simulink model "AERO421_FP4"  (R2024b)
settings: Solver=ode45  StartTime=0.0  StopTime=tspan  RelTol=1e-8  AbsTol=1e-8
model workspace (MATLAB code in the model file):
  | mu = 398601; % km
  | Re = 6378.137; %km
values from neighbouring files (symbols this model uses):
  E_b_ECI_0 = C2EulerAngles(C_b_ECI_0)    [AERO421_FP4_RJF_SR.m]
  E_b_LVLH_0 = [phi_0; theta_0; psi_0]    [AERO421_FP4_RJF_SR.m]
  q_b_ECI_0 = rotm2quat(C_b_ECI_0)    [AERO421_FP4_RJF_SR.m]
  q_b_LVLH_0 = [0; 0; 0; 1]    [AERO421_FP4_RJF_SR.m]
  T_c = [0; 0; 0]    [AERO421_FP4_RJF_SR.m]
  w_b_ECI_0 = [0.001; -0.001; 0.002]    [AERO421_FP4_RJF_SR.m]
undefined symbols (not defined in the file or in its folder): J, r_ECI_0, v_ECI_0
settings Model: Creator=emehiel  LastModifiedBy=rosha
settings SolverCC: AlgebraicLoopSolver=TrustRegion
settings DebuggingCC: UnconnectedInputMsg=warning  UnconnectedOutputMsg=warning  UnconnectedLineMsg=warning
settings ModelReferenceCC: EnableRefExpFcnMdlSchedulingChecks=on
settings RTWCC: GPUComputeCapability=3.5

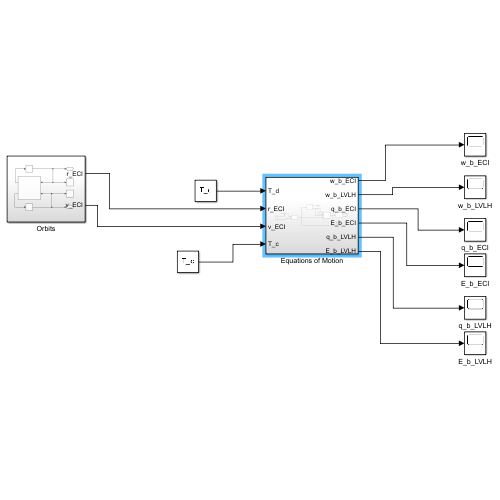
[thumbnail: Simulink's stored preview of the top-level diagram]
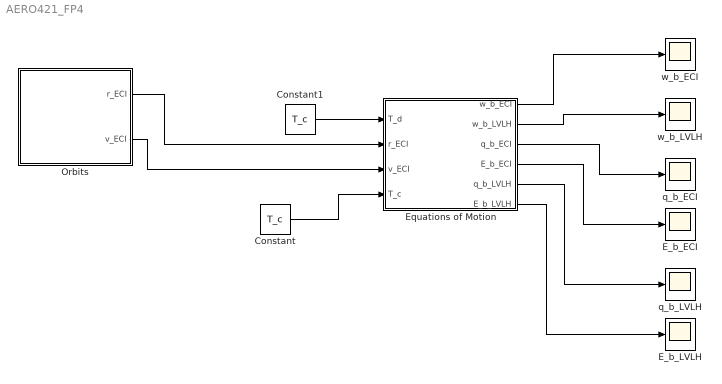
== system AERO421_FP4 ==
  Constant : Constant  Value=T_c
  Constant1 : Constant  Value=T_c
  E_b_ECI : Scope
  E_b_LVLH : Scope
  Equations of Motion : Subsystem
  Orbits : Subsystem
  q_b_ECI : Scope
  q_b_LVLH : Scope
  w_b_ECI : Scope
  w_b_LVLH : Scope
  wires:
  Orbits/1(r_ECI) -> Equations of Motion/2(r_ECI)
  Equations of Motion/3(q_b_ECI) -> q_b_ECI/1
  Equations of Motion/1(w_b_ECI) -> w_b_ECI/1
  Equations of Motion/4(E_b_ECI) -> E_b_ECI/1
  Equations of Motion/2(w_b_LVLH) -> w_b_LVLH/1
  Equations of Motion/5(q_b_LVLH) -> q_b_LVLH/1
  Equations of Motion/6(E_b_LVLH) -> E_b_LVLH/1
  Orbits/2(v_ECI) -> Equations of Motion/3(v_ECI)
  Constant/1 -> Equations of Motion/4(T_c)
  Constant1/1 -> Equations of Motion/1(T_d)

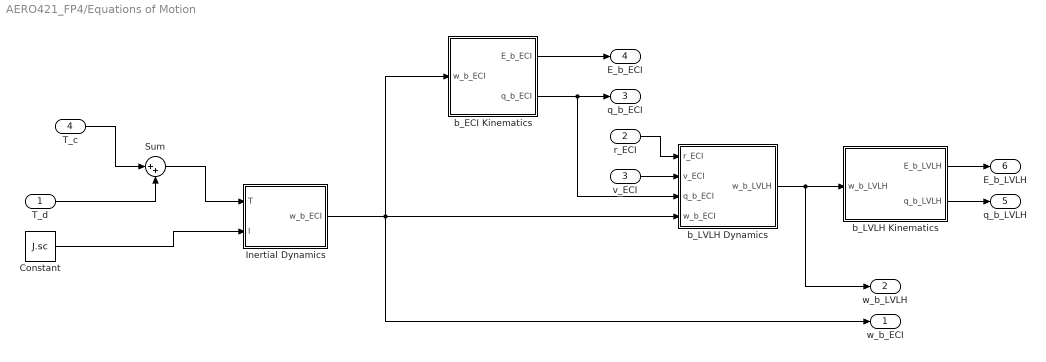
== system AERO421_FP4/Equations of Motion ==
  T_d : Inport
  r_ECI : Inport  Port=2
  v_ECI : Inport  Port=3
  T_c : Inport  Port=4
  Constant : Constant  Value=J.sc
  Inertial Dynamics : Subsystem
  Sum : Sum  Inputs=|++
  b_ECI Kinematics : Subsystem
  b_LVLH Dynamics : Subsystem
  b_LVLH Kinematics : Subsystem
  w_b_ECI : Outport  VectorParamsAs1DForOutWhenUnconnected=off
  w_b_LVLH : Outport  Port=2  PortDimensions=[3 1]  VectorParamsAs1DForOutWhenUnconnected=off
  q_b_ECI : Outport  Port=3  PortDimensions=[4 1]  VectorParamsAs1DForOutWhenUnconnected=off
  E_b_ECI : Outport  Port=4  PortDimensions=[3 1]  VectorParamsAs1DForOutWhenUnconnected=off
  q_b_LVLH : Outport  Port=5  PortDimensions=[4 1]  VectorParamsAs1DForOutWhenUnconnected=off
  E_b_LVLH : Outport  Port=6  PortDimensions=[3 1]  VectorParamsAs1DForOutWhenUnconnected=off
  wires:
  b_ECI Kinematics/1(E_b_ECI) -> E_b_ECI/1
  Constant/1 -> Inertial Dynamics/2(I)
  b_LVLH Kinematics/1(E_b_LVLH) -> E_b_LVLH/1
  Inertial Dynamics/1(w_b_ECI) -> w_b_ECI/1, b_ECI Kinematics/1(w_b_ECI), b_LVLH Dynamics/4(w_b_ECI)
  b_ECI Kinematics/2(q_b_ECI) -> b_LVLH Dynamics/3(q_b_ECI), q_b_ECI/1
  b_LVLH Kinematics/2(q_b_LVLH) -> q_b_LVLH/1
  r_ECI/1 -> b_LVLH Dynamics/1("r_ECI ")
  v_ECI/1 -> b_LVLH Dynamics/2(v_ECI)
  b_LVLH Dynamics/1(w_b_LVLH) -> w_b_LVLH/1, b_LVLH Kinematics/1(w_b_LVLH)
  T_d/1 -> Sum/2
  T_c/1 -> Sum/1
  Sum/1 -> Inertial Dynamics/1(T)

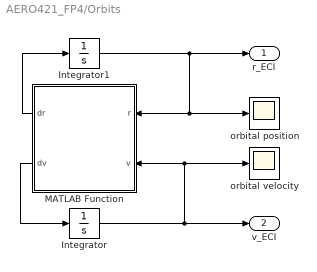
== system AERO421_FP4/Orbits ==
  Integrator : Integrator  InitialCondition=v_ECI_0
  Integrator1 : Integrator  InitialCondition=r_ECI_0
  MATLAB Function : MATLAB Function  TreatAsAtomicUnit=on
  orbital position : Scope
  orbital velocity : Scope
  r_ECI : Outport  VectorParamsAs1DForOutWhenUnconnected=off
  v_ECI : Outport  Port=2  VectorParamsAs1DForOutWhenUnconnected=off
  wires:
  Integrator/1 -> orbital velocity/1, MATLAB Function/2(v), v_ECI/1
  Integrator1/1 -> orbital position/1, MATLAB Function/1(r), r_ECI/1
  MATLAB Function/1(dr) -> Integrator1/1
  MATLAB Function/2(dv) -> Integrator/1

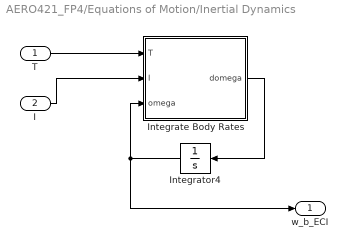
== system AERO421_FP4/Equations of Motion/Inertial Dynamics ==
  T : Inport
  I : Inport  Port=2
  Integrate Body Rates : MATLAB Function  TreatAsAtomicUnit=on
  Integrator4 : Integrator  InitialCondition=w_b_ECI_0
  w_b_ECI : Outport  VectorParamsAs1DForOutWhenUnconnected=off
  wires:
  Integrate Body Rates/1(domega) -> Integrator4/1
  I/1 -> Integrate Body Rates/2(I)
  T/1 -> Integrate Body Rates/1(T)
  Integrator4/1 -> w_b_ECI/1, Integrate Body Rates/3(omega)

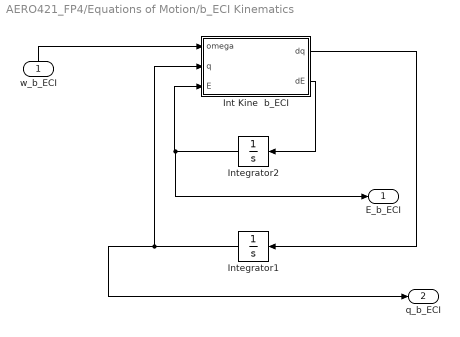
== system AERO421_FP4/Equations of Motion/b_ECI Kinematics ==
  w_b_ECI : Inport
  Int Kine  b_ECI : MATLAB Function  TreatAsAtomicUnit=on
  Integrator1 : Integrator  InitialCondition=q_b_ECI_0
  Integrator2 : Integrator  InitialCondition=E_b_ECI_0
  E_b_ECI : Outport  PortDimensions=[3 1]  VectorParamsAs1DForOutWhenUnconnected=off
  q_b_ECI : Outport  Port=2  PortDimensions=[4 1]  VectorParamsAs1DForOutWhenUnconnected=off
  wires:
  w_b_ECI/1 -> Int Kine  b_ECI/1(omega)
  Int Kine  b_ECI/1(dq) -> Integrator1/1
  Int Kine  b_ECI/2(dE) -> Integrator2/1
  Integrator1/1 -> q_b_ECI/1, Int Kine  b_ECI/2(q)
  Integrator2/1 -> E_b_ECI/1, Int Kine  b_ECI/3(E)

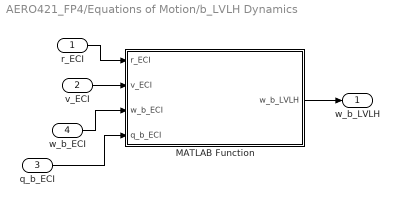
== system AERO421_FP4/Equations of Motion/b_LVLH Dynamics ==
  "r_ECI " : Inport
  v_ECI : Inport  Port=2
  q_b_ECI : Inport  Port=3
  w_b_ECI : Inport  Port=4
  MATLAB Function : MATLAB Function  TreatAsAtomicUnit=on
  w_b_LVLH : Outport  VectorParamsAs1DForOutWhenUnconnected=off
  wires:
  MATLAB Function/1(w_b_LVLH) -> w_b_LVLH/1
  "r_ECI "/1 -> MATLAB Function/1(r_ECI)
  v_ECI/1 -> MATLAB Function/2(v_ECI)
  q_b_ECI/1 -> MATLAB Function/4(q_b_ECI)
  w_b_ECI/1 -> MATLAB Function/3(w_b_ECI)

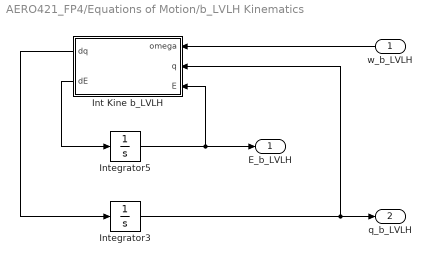
== system AERO421_FP4/Equations of Motion/b_LVLH Kinematics ==
  w_b_LVLH : Inport
  Int Kine b_LVLH : MATLAB Function  TreatAsAtomicUnit=on
  Integrator3 : Integrator  InitialCondition=q_b_LVLH_0
  Integrator5 : Integrator  InitialCondition=E_b_LVLH_0
  E_b_LVLH : Outport  PortDimensions=[3 1]  VectorParamsAs1DForOutWhenUnconnected=off
  q_b_LVLH : Outport  Port=2  VectorParamsAs1DForOutWhenUnconnected=off
  wires:
  Int Kine b_LVLH/1(dq) -> Integrator3/1
  Integrator3/1 -> Int Kine b_LVLH/2(q), q_b_LVLH/1
  Int Kine b_LVLH/2(dE) -> Integrator5/1
  Integrator5/1 -> E_b_LVLH/1, Int Kine b_LVLH/3(E)
  w_b_LVLH/1 -> Int Kine b_LVLH/1(omega)

== matlab function AERO421_FP4/Equations of Motion/Inertial Dynamics/Integrate Body Rates ==
  data: T input; I input; omega input; domega output
function domega = dynamics(T, I, omega)
%#codegen

domega = I\(T - cross(omega, I*omega));

== matlab function AERO421_FP4/Equations of Motion/b_ECI Kinematics/Int Kine  b_ECI ==
  data: omega input; q input; dq output; E input; dE output
function [dq,dE] = kinematics(omega, q, E)
%#codegen

% unpack quaternion

epsilon = q(1:3,1);
eta = q(4,1);

depsilon = 1/2*(eta*eye(3) + vcross(epsilon))*omega;
deta = -1/2*epsilon'*omega;

dq = [depsilon; deta];

LBI = 1/cos(E(2))*[cos(E(2)) sin(E(1))*sin(E(2))  cos(E(1))*sin(E(2));
                   0         cos(E(1))*cos(E(2)) -sin(E(1))*cos(E(2));
                   0         sin(E(1))            cos(E(1))];

dE = LBI*omega;

== matlab function AERO421_FP4/Orbits/MATLAB Function ==
  data: r input; dr output; v input; dv output
function [dr,dv] = orbitalDynamics(r, v)
%#codegen

mu = 398601; % km^3/s^2

dr = v;
dv = -mu*r/norm(r)^3;

== matlab function AERO421_FP4/Equations of Motion/b_LVLH Dynamics/MATLAB Function ==
  data: r_ECI input; v_ECI input; w_b_ECI input; q_b_ECI input; w_b_LVLH output
function w_b_LVLH = fcn(r_ECI, v_ECI, w_b_ECI, q_b_ECI)
%#codegen

% Compute the angular velocity of LVLH wrt ECI in Body components

Z_lvlh = -r_ECI/norm(r_ECI);
Y_lvlh = -cross(r_ECI,v_ECI)/norm(cross(r_ECI,v_ECI));
X_lvlh = cross(Y_lvlh,Z_lvlh);

C_LVLH_ECI = [X_lvlh,Y_lvlh,Z_lvlh];

w_LVLH_ECI = cross(r_ECI,v_ECI) / norm(r_ECI)^2;

% Initial Euler angles relating F_body and F_LVLH (given)???

eulZYX = quat2eul(q_b_ECI');

phi = eulZYX(3);
theta = eulZYX(2);
psi = eulZYX(1);

C_b_LVLH = rotx(rad2deg(phi))'*roty(rad2deg(theta))'*rotz(rad2deg(psi))';
C_b_ECI = C_b_LVLH*C_LVLH_ECI;


w_b_LVLH = w_b_ECI - C_b_ECI*w_LVLH_ECI;

== matlab function AERO421_FP4/Equations of Motion/b_LVLH Kinematics/Int Kine b_LVLH ==
  data: omega input; q input; dq output; E input; dE output
function [dq, dE] = kinematics(omega, q, E)
%#codegen

% unpack quaternion

q1 = q(1);
q2 = q(2);
q3 = q(3);
epsilon = [q1,q2,q3];
epsilonX = vcross(epsilon);
n = q(4);

% unpack euler

phi = E(1);
theta = E(2);
psi = E(3);

% compute the derivative of the quaternion components here

ndot = -0.5.*(epsilon)*omega;
epsilonDot = 0.5*(n*eye(3) + epsilonX)*omega;
dq = [epsilonDot;ndot];

% compute the derivative of the Euler Angle components here

rotm = [1,     sin(phi)*tan(theta), cos(phi)*tan(theta)
        0,     cos(phi),            -sin(phi)
        0,     sin(phi)*sec(theta), cos(phi)*sec(theta)];

dE = rotm*omega;
